simulink model "Twotanks_m71"  (R2020b)
settings: Solver=FixedStepAuto  StartTime=0.0  StopTime=300  FixedStep=0.1  RelTol=1e-3  EnableMultiTasking=on
model workspace (MAT data in the model file):
  F = [0; 0]
  Global = [3707764736; 2; 1; 1; 1; 1]
  InputSize = 5
  Operation = 'value'
  X = [1.91912110987  0.7189344389; 0.667300428728  0.319032887648; 0.539327875678  0.291550549769; 1.11428719774  0.782058235411; 0.458496889769  0.886118463221]
  cs : handle (value not decoded)
  curPath = '/Users/ceren.gebizli/Desktop/Shiva/QRA-Search/QRA-Search/Problems/SimulinkTesting'
  ext = ''
  generatedFile = '/Users/khouloud.gaaloul/Documents/Projects/SOCRaTeS/socrates/software/scalability/Simulink_Models/Twotanks/Twotanks_Model'
  hws = [3707764736; 2; 1; 1; 1; 1]
  input = [1.91912110987  0.7189344389; 0.667300428728  0.319032887648; 0.539327875678  0.291550549769; 1.11428719774  0.782058235411; 0.458496889769  0.886118463221]
  inputSize = 1
  j = 2
  m = matlab.io.MatFile
  m.Properties = matlab.io.matfile.Properties
  m.Properties.SupportsPartialAccess = 0
  m.Properties.Source = '/Users/khouloud.gaaloul/Documents/Projects/SOCRaTeS/socrates/software/scalability/RQ3/testcases/twotanks_tc_1.mat'
  matfilename = 'twotanks_tc_1.mat'
  model_cs : handle (value not decoded)
  modelpath = '/Users/khouloud.gaaloul/Documents/Projects/SOCRaTeS/socrates/software/scalability/Simulink_Models/Twotanks/'
  name = 'Twotanks_Model'
  nbrInputs = 2
  nbrTimeSteps = 5001
  p = 1
  path = '/Users/khouloud.gaaloul/Documents/Projects/SOCRaTeS/socrates/software/scalability/Simulink_Models/Twotanks'
  pr.model_name = 'Twotanks_Model'
  pr.fc = 5000
  pr.stime = 500
  problem : object (value not decoded)
  problems = {'twotanks'}
  tank1_init_height_m = 1.91912110987
  tank2_init_height_m = 0.7189344389
  testcase.signal = [0.0460270741829 0.899426437102]
  timestep = 2
  var.signal = [0.0460270741829 0.899426437102]
undefined symbols (not defined in the file): tank1_cross_section_area_m2_in, tank1_pump_flow_rate_m3s_in, tank1_sensor_hi_height_m_in, tank1_sensor_lo_height_m_in, tank1_valve_flow_rate_m3s_in, tank2_cross_section_area_m2_in, tank2_e_valve_flow_rate_m3s_in, tank2_p_valve_flow_rate_m3s_in, tank2_sensor_hi_height_m_in, tank2_sensor_lo_height_m_in, tank2_sensor_md_height_m_in
libraries: simulink x12
settings Model: Creator=Kerianne  LastModifiedBy=Xiao Ling
settings DataIOCC: ExternalInput=var  SaveFormat=StructureWithTime  SignalLoggingSaveFormat=ModelDataLogs  ReturnWorkspaceOutputs=off  OutputSaveName=varout  LoggingToFile=on
settings OptimizationCC: DefaultParameterBehavior=Inlined  ExpressionDepthLimit=2147483647  LifeSpan=inf
settings DebuggingCC: UnderspecifiedInitializationDetection=Classic  MergeDetectMultiDrivingBlocksExec=none  SolverPrmCheckMsg=warning  MultiTaskDSMMsg=warning  MultiTaskCondExecSysMsg=none  StateNameClashWarn=warning  SFUnexpectedBacktrackingDiag=warning  SFNoUnconditionalDefaultTransitionDiag=warning  SFExecutionAtInitializationDiag=none  ArithmeticOperatorsInVariantConditions=warning
settings HardwareCC: ProdBitPerPointer=32  ProdBitPerSizeT=32  ProdBitPerPtrDiffT=32  ProdLargestAtomicFloat=None  ProdIntDivRoundTo=Undefined  ProdEndianess=Unspecified  ProdWordSize=32  ProdHWDeviceType=32-bit Generic
settings ModelReferenceCC: PropagateSignalLabelsOutOfModel=off
settings SFSimCC: SimUseLocalCustomCode=off  CustomCodeUndefinedFunction=UseInterfaceOnly
settings RTWCC: RTWUseLocalCustomCode=off
settings CodeAppCC: StateflowObjectComments=on
settings GRTTargetCC: TargetLangStandard=C89/C90 (ANSI)
settings ConfigComp: CovMetricSettings=dw  CovSaveCumulativeToWorkspaceVar=on  CovSaveSingleToWorkspaceVar=on  CovExternalEMLEnable=off

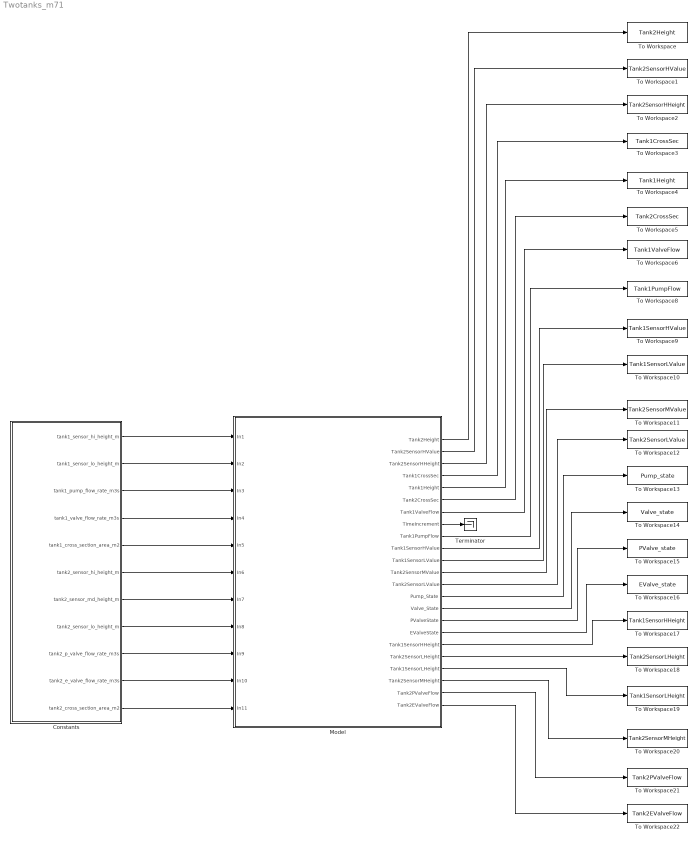
== system Twotanks_m71 ==
  Constants : Subsystem
  Model : Subsystem
  Terminator : Terminator
  To Workspace : ToWorkspace  VariableName=Tank2Height  SampleTime=-1
  To Workspace1 : ToWorkspace  VariableName=Tank2SensorHValue  SampleTime=-1
  To Workspace10 : ToWorkspace  VariableName=Tank1SensorLValue  SampleTime=-1
  To Workspace11 : ToWorkspace  VariableName=Tank2SensorMValue  SampleTime=-1
  To Workspace12 : ToWorkspace  VariableName=Tank2SensorLValue  SampleTime=-1
  To Workspace13 : ToWorkspace  VariableName=Pump_state  SampleTime=-1
  To Workspace14 : ToWorkspace  VariableName=Valve_state  SampleTime=-1
  To Workspace15 : ToWorkspace  VariableName=PValve_state  SampleTime=-1
  To Workspace16 : ToWorkspace  VariableName=EValve_state  SampleTime=-1
  To Workspace17 : ToWorkspace  VariableName=Tank1SensorHHeight  SampleTime=-1
  To Workspace18 : ToWorkspace  VariableName=Tank2SensorLHeight  SampleTime=-1
  To Workspace19 : ToWorkspace  VariableName=Tank1SensorLHeight  SampleTime=-1
  To Workspace2 : ToWorkspace  VariableName=Tank2SensorHHeight  SampleTime=-1
  To Workspace20 : ToWorkspace  VariableName=Tank2SensorMHeight  SampleTime=-1
  To Workspace21 : ToWorkspace  VariableName=Tank2PValveFlow  SampleTime=-1
  To Workspace22 : ToWorkspace  VariableName=Tank2EValveFlow  SampleTime=-1
  To Workspace3 : ToWorkspace  VariableName=Tank1CrossSec  SampleTime=-1
  To Workspace4 : ToWorkspace  VariableName=Tank1Height  SampleTime=-1
  To Workspace5 : ToWorkspace  VariableName=Tank2CrossSec  SampleTime=-1
  To Workspace6 : ToWorkspace  VariableName=Tank1ValveFlow  SampleTime=-1
  To Workspace8 : ToWorkspace  VariableName=Tank1PumpFlow  SampleTime=-1
  To Workspace9 : ToWorkspace  VariableName=Tank1SensorHValue  SampleTime=-1
  wires:
  Constants/1(tank1_sensor_hi_height_m) -> Model/1(In1)
  Constants/2(tank1_sensor_lo_height_m) -> Model/2(In2)
  Constants/3(tank1_pump_flow_rate_m3s) -> Model/3(In3)
  Constants/4(tank1_valve_flow_rate_m3s) -> Model/4(In4)
  Constants/5(tank1_cross_section_area_m2) -> Model/5(In5)
  Constants/6(tank2_sensor_hi_height_m) -> Model/6(In6)
  Constants/7(tank2_sensor_md_height_m) -> Model/7(In7)
  Constants/8(tank2_sensor_lo_height_m) -> Model/8(In8)
  Constants/9(tank2_p_valve_flow_rate_m3s) -> Model/9(In9)
  Constants/10(tank2_e_valve_flow_rate_m3s) -> Model/10(In10)
  Constants/11(tank2_cross_section_area_m2) -> Model/11(In11)
  Model/1(Tank2Height) -> To Workspace/1
  Model/2(Tank2SensorHValue) -> To Workspace1/1
  Model/3(Tank2SensorHHeight) -> To Workspace2/1
  Model/7(Tank1ValveFlow) -> To Workspace6/1
  Model/8(TimeIncrement) -> Terminator/1
  Model/6(Tank2CrossSec) -> To Workspace5/1
  Model/5(Tank1Height) -> To Workspace4/1
  Model/9(Tank1PumpFlow) -> To Workspace8/1
  Model/10(Tank1SensorHValue) -> To Workspace9/1
  Model/11(Tank1SensorLValue) -> To Workspace10/1
  Model/12(Tank2SensorMValue) -> To Workspace11/1
  Model/13(Tank2SensorLValue) -> To Workspace12/1
  Model/16(PValveState) -> To Workspace15/1
  Model/15(Valve_State) -> To Workspace14/1
  Model/14(Pump_State) -> To Workspace13/1
  Model/19(Tank2SensorLHeight) -> To Workspace18/1
  Model/18(Tank1SensorHHeight) -> To Workspace17/1
  Model/17(EValveState) -> To Workspace16/1
  Model/20(Tank1SensorLHeight) -> To Workspace19/1
  Model/21(Tank2SensorMHeight) -> To Workspace20/1
  Model/23(Tank2EValveFlow) -> To Workspace22/1
  Model/22(Tank2PValveFlow) -> To Workspace21/1
  Model/4(Tank1CrossSec) -> To Workspace3/1

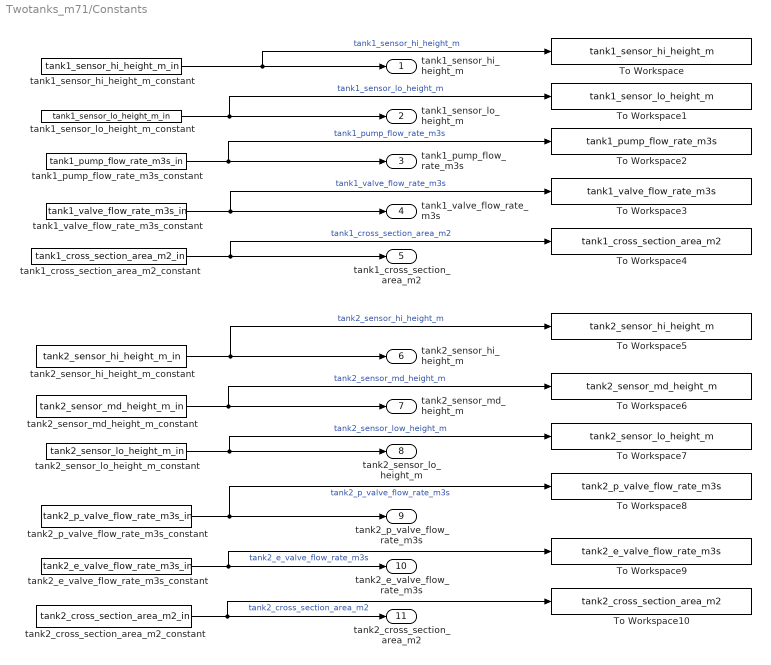
== system Twotanks_m71/Constants ==
  To Workspace : ToWorkspace  VariableName=tank1_sensor_hi_height_m  SampleTime=-1
  To Workspace1 : ToWorkspace  VariableName=tank1_sensor_lo_height_m  SampleTime=-1
  To Workspace10 : ToWorkspace  VariableName=tank2_cross_section_area_m2  SampleTime=-1
  To Workspace2 : ToWorkspace  VariableName=tank1_pump_flow_rate_m3s  SampleTime=-1
  To Workspace3 : ToWorkspace  VariableName=tank1_valve_flow_rate_m3s  SampleTime=-1
  To Workspace4 : ToWorkspace  VariableName=tank1_cross_section_area_m2  SampleTime=-1
  To Workspace5 : ToWorkspace  VariableName=tank2_sensor_hi_height_m  SampleTime=-1
  To Workspace6 : ToWorkspace  VariableName=tank2_sensor_md_height_m  SampleTime=-1
  To Workspace7 : ToWorkspace  VariableName=tank2_sensor_lo_height_m  SampleTime=-1
  To Workspace8 : ToWorkspace  VariableName=tank2_p_valve_flow_rate_m3s  SampleTime=-1
  To Workspace9 : ToWorkspace  VariableName=tank2_e_valve_flow_rate_m3s  SampleTime=-1
  tank1_cross_section_area_m2_constant : Constant  Value=tank1_cross_section_area_m2_in
  tank1_pump_flow_rate_m3s_constant : Constant  Value=tank1_pump_flow_rate_m3s_in
  tank1_sensor_hi_height_m_constant : Constant  Value=tank1_sensor_hi_height_m_in
  tank1_sensor_lo_height_m_constant : Constant  Value=tank1_sensor_lo_height_m_in
  tank1_valve_flow_rate_m3s_constant : Constant  Value=tank1_valve_flow_rate_m3s_in
  tank2_cross_section_area_m2_constant : Constant  Value=tank2_cross_section_area_m2_in
  tank2_e_valve_flow_rate_m3s_constant : Constant  Value=tank2_e_valve_flow_rate_m3s_in
  tank2_p_valve_flow_rate_m3s_constant : Constant  Value=tank2_p_valve_flow_rate_m3s_in
  tank2_sensor_hi_height_m_constant : Constant  Value=tank2_sensor_hi_height_m_in
  tank2_sensor_lo_height_m_constant : Constant  Value=tank2_sensor_lo_height_m_in
  tank2_sensor_md_height_m_constant : Constant  Value=tank2_sensor_md_height_m_in
  tank1_sensor_hi_height_m : Outport  VectorParamsAs1DForOutWhenUnconnected=off
  tank1_sensor_lo_height_m : Outport  Port=2  VectorParamsAs1DForOutWhenUnconnected=off
  tank1_pump_flow_rate_m3s : Outport  Port=3  VectorParamsAs1DForOutWhenUnconnected=off
  tank1_valve_flow_rate_m3s : Outport  Port=4  VectorParamsAs1DForOutWhenUnconnected=off
  tank1_cross_section_area_m2 : Outport  Port=5  VectorParamsAs1DForOutWhenUnconnected=off
  tank2_sensor_hi_height_m : Outport  Port=6  VectorParamsAs1DForOutWhenUnconnected=off
  tank2_sensor_md_height_m : Outport  Port=7  VectorParamsAs1DForOutWhenUnconnected=off
  tank2_sensor_lo_height_m : Outport  Port=8  VectorParamsAs1DForOutWhenUnconnected=off
  tank2_p_valve_flow_rate_m3s : Outport  Port=9  VectorParamsAs1DForOutWhenUnconnected=off
  tank2_e_valve_flow_rate_m3s : Outport  Port=10  VectorParamsAs1DForOutWhenUnconnected=off
  tank2_cross_section_area_m2 : Outport  Port=11  VectorParamsAs1DForOutWhenUnconnected=off
  wires:
  tank2_sensor_hi_height_m_constant/1 -> To Workspace5/1, tank2_sensor_hi_height_m/1  "tank2_sensor_hi_height_m"
  tank2_sensor_lo_height_m_constant/1 -> To Workspace7/1, tank2_sensor_lo_height_m/1  "tank2_sensor_low_height_m"
  tank1_sensor_hi_height_m_constant/1 -> To Workspace/1, tank1_sensor_hi_height_m/1  "tank1_sensor_hi_height_m"
  tank1_pump_flow_rate_m3s_constant/1 -> tank1_pump_flow_rate_m3s/1, To Workspace2/1  "tank1_pump_flow_rate_m3s"
  tank1_cross_section_area_m2_constant/1 -> To Workspace4/1, tank1_cross_section_area_m2/1  "tank1_cross_section_area_m2"
  tank1_valve_flow_rate_m3s_constant/1 -> To Workspace3/1, tank1_valve_flow_rate_m3s/1  "tank1_valve_flow_rate_m3s"
  tank1_sensor_lo_height_m_constant/1 -> tank1_sensor_lo_height_m/1, To Workspace1/1  "tank1_sensor_lo_height_m"
  tank2_p_valve_flow_rate_m3s_constant/1 -> tank2_p_valve_flow_rate_m3s/1, To Workspace8/1  "tank2_p_valve_flow_rate_m3s"
  tank2_cross_section_area_m2_constant/1 -> To Workspace10/1, tank2_cross_section_area_m2/1  "tank2_cross_section_area_m2"
  tank2_e_valve_flow_rate_m3s_constant/1 -> To Workspace9/1, tank2_e_valve_flow_rate_m3s/1  "tank2_e_valve_flow_rate_m3s"
  tank2_sensor_md_height_m_constant/1 -> To Workspace6/1, tank2_sensor_md_height_m/1  "tank2_sensor_md_height_m"

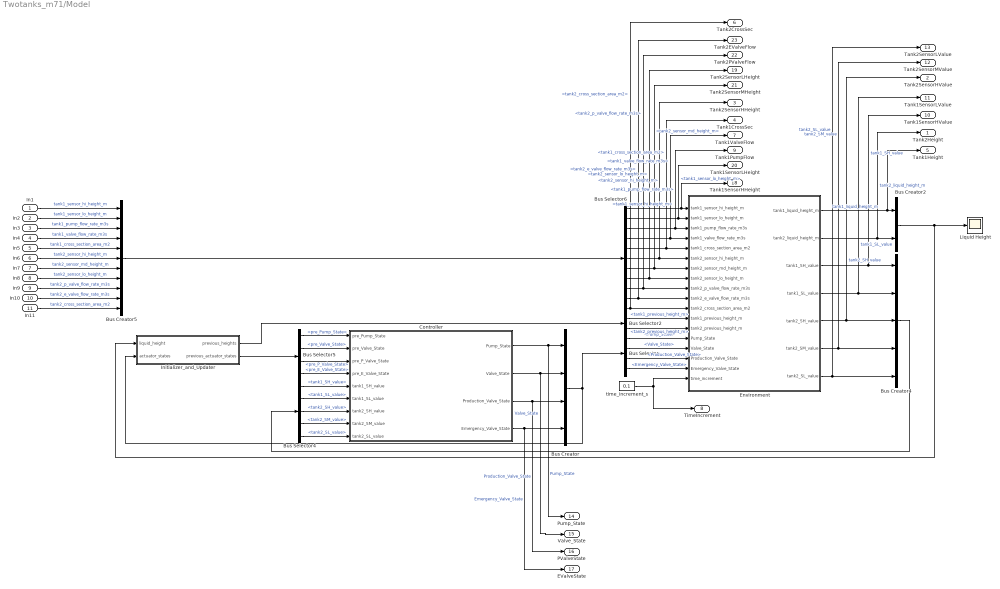
== system Twotanks_m71/Model ==
  In1 : Inport
  In2 : Inport  Port=2
  In3 : Inport  Port=3
  In4 : Inport  Port=4
  In5 : Inport  Port=5
  In6 : Inport  Port=6
  In7 : Inport  Port=7
  In8 : Inport  Port=8
  In9 : Inport  Port=9
  In10 : Inport  Port=10
  In11 : Inport  Port=11
  Bus Creator : BusCreator  Inputs=4
  Bus Creator2 : BusCreator  Inputs='tank1_liquid_height_m','tank2_liquid_height_m'
  Bus Creator4 : BusCreator  Inputs='tank1_SH_value','tank1_SL_value','tank2_SH_value','tank2_SM_value','tank2_SL_value'
  Bus Creator5 : BusCreator  Inputs='tank1_sensor_hi_height_m','tank1_sensor_lo_height_m','tank1_pump_flow_rate_m3s','tank1_valve_flow_rate_m3s','tank1_cross_section_area_m2','tank2_sensor_hi_height_m','tank2_sensor_md_height_m','tank2_sensor_lo_height_m','tank2_p_valve_flow_rate_m3s','tank2_e_valve_flow_rate_m3s','tank2_cross_section_area_m2'
  Bus Selector : BusSelector  OutputSignals=Pump_State,Valve_State,Production_Valve_State,Emergency_Valve_State
  Bus Selector2 : BusSelector  OutputSignals=tank1_previous_height_m,tank2_previous_height_m
  Bus Selector4 : BusSelector  OutputSignals=tank1_SH_value,tank1_SL_value,tank2_SH_value,tank2_SM_value,tank2_SL_value
  Bus Selector5 : BusSelector  OutputSignals=pre_Pump_State,pre_Valve_State,pre_P_Valve_State,pre_E_Valve_State
  Bus Selector6 : BusSelector  OutputSignals=tank1_sensor_hi_height_m,tank1_sensor_lo_height_m,tank1_pump_flow_rate_m3s,tank1_valve_flow_rate_m3s,tank1_cross_section_area_m2,tank2_sensor_hi_height_m,tank2_sensor_md_height_m,tank2_sensor_lo_height_m,tank2_p_valve_flow_rate_m3s,tank2_e_valve_flow_rate_m3s,tank2_cross_section_area_m2
  Controller : Subsystem
  Environment : Subsystem
  Initializer_and_Updater : Subsystem
  Liquid Height : Scope
  time_increment_s : Constant  Value=0.1
  Tank2Height : Outport  VectorParamsAs1DForOutWhenUnconnected=off
  Tank2SensorHValue : Outport  Port=2  VectorParamsAs1DForOutWhenUnconnected=off
  Tank2SensorHHeight : Outport  Port=3  VectorParamsAs1DForOutWhenUnconnected=off
  Tank1CrossSec : Outport  Port=4  VectorParamsAs1DForOutWhenUnconnected=off
  Tank1Height : Outport  Port=5  VectorParamsAs1DForOutWhenUnconnected=off
  Tank2CrossSec : Outport  Port=6  VectorParamsAs1DForOutWhenUnconnected=off
  Tank1ValveFlow : Outport  Port=7  VectorParamsAs1DForOutWhenUnconnected=off
  TimeIncrement : Outport  Port=8  VectorParamsAs1DForOutWhenUnconnected=off
  Tank1PumpFlow : Outport  Port=9  VectorParamsAs1DForOutWhenUnconnected=off
  Tank1SensorHValue : Outport  Port=10  VectorParamsAs1DForOutWhenUnconnected=off
  Tank1SensorLValue : Outport  Port=11  VectorParamsAs1DForOutWhenUnconnected=off
  Tank2SensorMValue : Outport  Port=12  VectorParamsAs1DForOutWhenUnconnected=off
  Tank2SensorLValue : Outport  Port=13  VectorParamsAs1DForOutWhenUnconnected=off
  Pump_State : Outport  Port=14  VectorParamsAs1DForOutWhenUnconnected=off
  Valve_State : Outport  Port=15  VectorParamsAs1DForOutWhenUnconnected=off
  PValveState : Outport  Port=16  VectorParamsAs1DForOutWhenUnconnected=off
  EValveState : Outport  Port=17  VectorParamsAs1DForOutWhenUnconnected=off
  Tank1SensorHHeight : Outport  Port=18  VectorParamsAs1DForOutWhenUnconnected=off
  Tank2SensorLHeight : Outport  Port=19  VectorParamsAs1DForOutWhenUnconnected=off
  Tank1SensorLHeight : Outport  Port=20  VectorParamsAs1DForOutWhenUnconnected=off
  Tank2SensorMHeight : Outport  Port=21  VectorParamsAs1DForOutWhenUnconnected=off
  Tank2PValveFlow : Outport  Port=22  VectorParamsAs1DForOutWhenUnconnected=off
  Tank2EValveFlow : Outport  Port=23  VectorParamsAs1DForOutWhenUnconnected=off
  wires:
  In8/1 -> Bus Creator5/8  "tank2_sensor_lo_height_m"
  Bus Selector6/7 -> Environment/7(tank2_sensor_md_height_m), Tank2SensorMHeight/1  "<tank2_sensor_md_height_m>"
  Initializer_and_Updater/1(previous_heights) -> Bus Selector2/1
  Bus Selector6/10 -> Environment/10(tank2_e_valve_flow_rate_m3s), Tank2EValveFlow/1  "<tank2_e_valve_flow_rate_m3s>"
  Bus Selector6/3 -> Tank1PumpFlow/1, Environment/3(tank1_pump_flow_rate_m3s)  "<tank1_pump_flow_rate_m3s>"
  Bus Selector5/1 -> Controller/1(pre_Pump_State)  "<pre_Pump_State>"
  Environment/1(tank1_liquid_height_m) -> Tank1Height/1, Bus Creator2/1  "tank1_liquid_height_m"
  Bus Selector6/1 -> Tank1SensorHHeight/1, Environment/1(tank1_sensor_hi_height_m)  "<tank1_sensor_hi_height_m>"
  Bus Selector4/3 -> Controller/7(tank2_SH_value)  "<tank2_SH_value>"
  Bus Selector5/3 -> Controller/3(pre_P_Valve_State)  "<pre_P_Valve_State>"
  Bus Selector4/2 -> Controller/6(tank1_SL_value)  "<tank1_SL_value>"
  In6/1 -> Bus Creator5/6  "tank2_sensor_hi_height_m"
  Bus Selector/2 -> Environment/15(Valve_State)  "<Valve_State>"
  time_increment_s/1 -> Environment/18(time_increment), TimeIncrement/1
  Bus Selector6/6 -> Tank2SensorHHeight/1, Environment/6(tank2_sensor_hi_height_m)  "<tank2_sensor_hi_height_m>"
  Bus Selector4/4 -> Controller/8(tank2_SM_value)  "<tank2_SM_value>"
  In1/1 -> Bus Creator5/1  "tank1_sensor_hi_height_m"
  Environment/6(tank2_SM_value) -> Bus Creator4/4, Tank2SensorMValue/1  "tank2_SM_value"
  In7/1 -> Bus Creator5/7  "tank2_sensor_md_height_m"
  Bus Selector4/1 -> Controller/5(tank1_SH_value)  "<tank1_SH_value>"
  Controller/4(Emergency_Valve_State) -> EValveState/1, Bus Creator/4  "Emergency_Valve_State"
  Bus Selector6/9 -> Environment/9(tank2_p_valve_flow_rate_m3s), Tank2PValveFlow/1  "<tank2_p_valve_flow_rate_m3s>"
  Bus Selector6/4 -> Environment/4(tank1_valve_flow_rate_m3s), Tank1ValveFlow/1  "<tank1_valve_flow_rate_m3s>"
  Bus Creator5/1 -> Bus Selector6/1
  In5/1 -> Bus Creator5/5  "tank1_cross_section_area_m2"
  In10/1 -> Bus Creator5/10  "tank2_e_valve_flow_rate_m3s"
  Bus Creator4/1 -> Bus Selector4/1
  Environment/2(tank2_liquid_height_m) -> Tank2Height/1, Bus Creator2/2  "tank2_liquid_height_m"
  Bus Selector6/8 -> Environment/8(tank2_sensor_lo_height_m), Tank2SensorLHeight/1  "<tank2_sensor_lo_height_m>"
  Bus Selector/4 -> Environment/17(Emergency_Valve_State)  "<Emergency_Valve_State>"
  Environment/4(tank1_SL_value) -> Bus Creator4/2, Tank1SensorLValue/1  "tank1_SL_value"
  Bus Selector/3 -> Environment/16(Production_Valve_State)  "<Production_Valve_State>"
  In2/1 -> Bus Creator5/2  "tank1_sensor_lo_height_m"
  Bus Selector4/5 -> Controller/9(tank2_SL_value)  "<tank2_SL_value>"
  Bus Selector/1 -> Environment/14(Pump_State)  "<Pump_State>"
  Bus Selector6/2 -> Environment/2(tank1_sensor_lo_height_m), Tank1SensorLHeight/1  "<tank1_sensor_lo_height_m>"
  Bus Selector6/5 -> Tank1CrossSec/1, Environment/5(tank1_cross_section_area_m2)  "<tank1_cross_section_area_m2>"
  Environment/3(tank1_SH_value) -> Tank1SensorHValue/1, Bus Creator4/1  "tank1_SH_value"
  Controller/2(Valve_State) -> Bus Creator/2, Valve_State/1  "Valve_State"
  In4/1 -> Bus Creator5/4  "tank1_valve_flow_rate_m3s"
  In11/1 -> Bus Creator5/11  "tank2_cross_section_area_m2"
  Initializer_and_Updater/2(previous_actuator_states) -> Bus Selector5/1
  Environment/5(tank2_SH_value) -> Bus Creator4/3, Tank2SensorHValue/1  "tank2_SH_value"
  Bus Selector5/2 -> Controller/2(pre_Valve_State)  "<pre_Valve_State>"
  Bus Selector2/1 -> Environment/12(tank1_previous_height_m)  "<tank1_previous_height_m>"
  Environment/7(tank2_SL_value) -> Bus Creator4/5, Tank2SensorLValue/1  "tank2_SL_value"
  Controller/3(Production_Valve_State) -> PValveState/1, Bus Creator/3  "Production_Valve_State"
  Controller/1(Pump_State) -> Bus Creator/1, Pump_State/1  "Pump_State"
  In3/1 -> Bus Creator5/3  "tank1_pump_flow_rate_m3s"
  Bus Creator/1 -> Bus Selector/1, Initializer_and_Updater/2(actuator_states)
  Bus Creator2/1 -> Initializer_and_Updater/1(liquid_height), Liquid Height/1
  Bus Selector6/11 -> Environment/11(tank2_cross_section_area_m2), Tank2CrossSec/1  "<tank2_cross_section_area_m2>"
  Bus Selector2/2 -> Environment/13(tank2_previous_height_m)  "<tank2_previous_height_m>"
  Bus Selector5/4 -> Controller/4(pre_E_Valve_State)  "<pre_E_Valve_State>"
  In9/1 -> Bus Creator5/9  "tank2_p_valve_flow_rate_m3s"

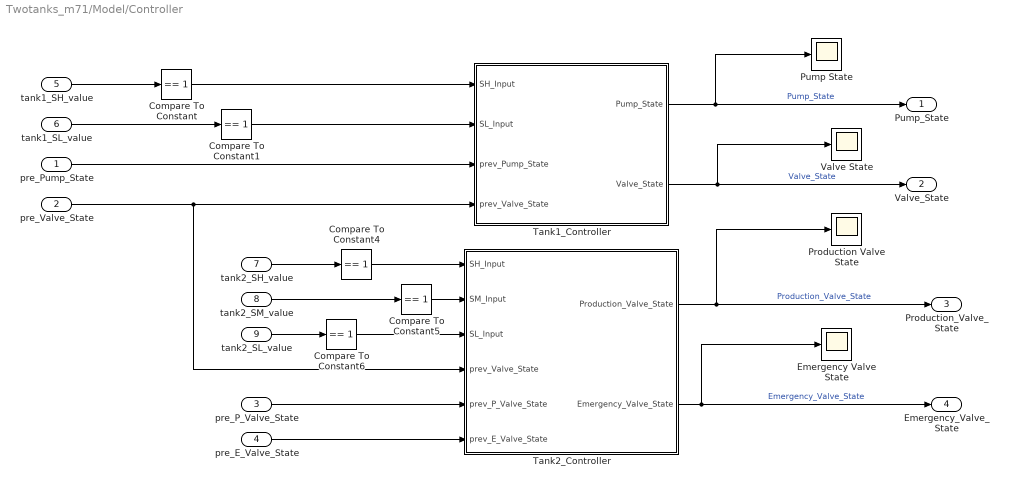
== system Twotanks_m71/Model/Controller ==
  pre_Pump_State : Inport
  pre_Valve_State : Inport  Port=2
  pre_P_Valve_State : Inport  Port=3
  pre_E_Valve_State : Inport  Port=4
  tank1_SH_value : Inport  Port=5
  tank1_SL_value : Inport  Port=6
  tank2_SH_value : Inport  Port=7
  tank2_SM_value : Inport  Port=8
  tank2_SL_value : Inport  Port=9
  Compare To Constant{,1,4..6} (5 alike) : simulink/Logic and Bit Operations/Compare To Constant  relop===  const=1  OutDataTypeStr=boolean
  Emergency Valve State : Scope
  Production Valve State : Scope
  "Pump State " : Scope
  Tank1_Controller : Subsystem
  Tank2_Controller : Subsystem
  Valve State : Scope
  Pump_State : Outport  VectorParamsAs1DForOutWhenUnconnected=off
  Valve_State : Outport  Port=2  VectorParamsAs1DForOutWhenUnconnected=off
  Production_Valve_State : Outport  Port=3  VectorParamsAs1DForOutWhenUnconnected=off
  Emergency_Valve_State : Outport  Port=4  VectorParamsAs1DForOutWhenUnconnected=off
  wires:
  tank1_SL_value/1 -> Compare To Constant1/1
  tank2_SL_value/1 -> Compare To Constant6/1
  pre_E_Valve_State/1 -> Tank2_Controller/6(prev_E_Valve_State)
  Compare To Constant1/1 -> Tank1_Controller/2(SL_Input)
  Tank1_Controller/1(Pump_State) -> Pump_State/1, "Pump State "/1  "Pump_State"
  Tank1_Controller/2(Valve_State) -> Valve_State/1, Valve State/1  "Valve_State"
  Compare To Constant/1 -> Tank1_Controller/1(SH_Input)
  pre_Pump_State/1 -> Tank1_Controller/3(prev_Pump_State)
  tank2_SH_value/1 -> Compare To Constant4/1
  Compare To Constant6/1 -> Tank2_Controller/3(SL_Input)
  Compare To Constant4/1 -> Tank2_Controller/1(SH_Input)
  tank1_SH_value/1 -> Compare To Constant/1
  pre_Valve_State/1 -> Tank2_Controller/4(prev_Valve_State), Tank1_Controller/4(prev_Valve_State)
  Tank2_Controller/2(Emergency_Valve_State) -> Emergency_Valve_State/1, Emergency Valve State/1  "Emergency_Valve_State"
  tank2_SM_value/1 -> Compare To Constant5/1
  Compare To Constant5/1 -> Tank2_Controller/2(SM_Input)
  Tank2_Controller/1(Production_Valve_State) -> Production_Valve_State/1, Production Valve State/1  "Production_Valve_State"
  pre_P_Valve_State/1 -> Tank2_Controller/5(prev_P_Valve_State)

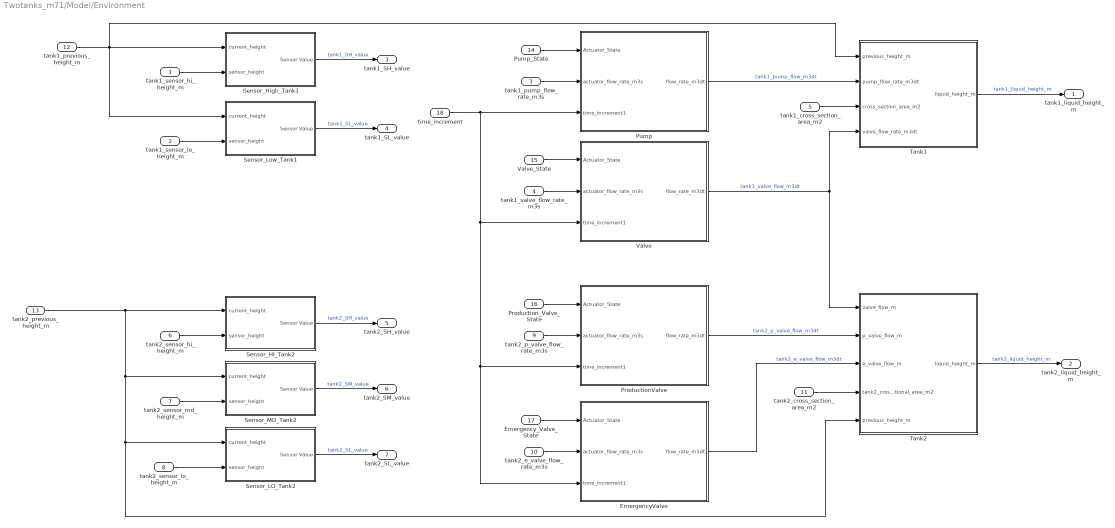
== system Twotanks_m71/Model/Environment ==
  tank1_sensor_hi_height_m : Inport
  tank1_sensor_lo_height_m : Inport  Port=2
  tank1_pump_flow_rate_m3s : Inport  Port=3
  tank1_valve_flow_rate_m3s : Inport  Port=4
  tank1_cross_section_area_m2 : Inport  Port=5
  tank2_sensor_hi_height_m : Inport  Port=6
  tank2_sensor_md_height_m : Inport  Port=7
  tank2_sensor_lo_height_m : Inport  Port=8
  tank2_p_valve_flow_rate_m3s : Inport  Port=9
  tank2_e_valve_flow_rate_m3s : Inport  Port=10
  tank2_cross_section_area_m2 : Inport  Port=11
  tank1_previous_height_m : Inport  Port=12
  tank2_previous_height_m : Inport  Port=13
  Pump_State : Inport  Port=14
  Valve_State : Inport  Port=15
  Production_Valve_State : Inport  Port=16
  Emergency_Valve_State : Inport  Port=17
  time_increment : Inport  Port=18
  EmergencyValve : Subsystem
  ProductionValve : Subsystem
  Pump : Subsystem
  Sensor_HI_Tank2 : Subsystem
  Sensor_High_Tank1 : Subsystem
  Sensor_LO_Tank2 : Subsystem
  Sensor_Low_Tank1 : Subsystem
  Sensor_MD_Tank2 : Subsystem
  Tank1 : Subsystem
  Tank2 : Subsystem
  Valve : Subsystem
  tank1_liquid_height_m : Outport  VectorParamsAs1DForOutWhenUnconnected=off
  tank2_liquid_height_m : Outport  Port=2  VectorParamsAs1DForOutWhenUnconnected=off
  tank1_SH_value : Outport  Port=3  VectorParamsAs1DForOutWhenUnconnected=off
  tank1_SL_value : Outport  Port=4  VectorParamsAs1DForOutWhenUnconnected=off
  tank2_SH_value : Outport  Port=5  VectorParamsAs1DForOutWhenUnconnected=off
  tank2_SM_value : Outport  Port=6  VectorParamsAs1DForOutWhenUnconnected=off
  tank2_SL_value : Outport  Port=7  VectorParamsAs1DForOutWhenUnconnected=off
  wires:
  Tank1/1(liquid_height_m) -> tank1_liquid_height_m/1  "tank1_liquid_height_m"
  time_increment/1 -> Pump/3(time_increment1), Valve/3(time_increment1), EmergencyValve/3(time_increment1), ProductionValve/3(time_increment1)
  tank2_sensor_hi_height_m/1 -> Sensor_HI_Tank2/2(sensor_height)
  Sensor_Low_Tank1/1(Sensor Value) -> tank1_SL_value/1  "tank1_SL_value"
  Sensor_HI_Tank2/1(Sensor Value) -> tank2_SH_value/1  "tank2_SH_value"
  Sensor_High_Tank1/1(Sensor Value) -> tank1_SH_value/1  "tank1_SH_value"
  tank1_pump_flow_rate_m3s/1 -> Pump/2(actuator_flow_rate_m3s)
  Sensor_LO_Tank2/1(Sensor Value) -> tank2_SL_value/1  "tank2_SL_value"
  tank2_sensor_lo_height_m/1 -> Sensor_LO_Tank2/2(sensor_height)
  tank1_valve_flow_rate_m3s/1 -> Valve/2(actuator_flow_rate_m3s)
  Sensor_MD_Tank2/1(Sensor Value) -> tank2_SM_value/1  "tank2_SM_value"
  tank2_p_valve_flow_rate_m3s/1 -> ProductionValve/2(actuator_flow_rate_m3s)
  tank2_previous_height_m/1 -> Sensor_HI_Tank2/1(current_height), Sensor_MD_Tank2/1(current_height), Sensor_LO_Tank2/1(current_height), Tank2/5(previous_height_m)
  EmergencyValve/1(flow_rate_m3dt) -> Tank2/3(e_valve_flow_m)  "tank2_e_valve_flow_m3dt"
  Pump/1(flow_rate_m3dt) -> Tank1/2(pump_flow_rate_m3dt)  "tank1_pump_flow_m3dt"
  Valve/1(flow_rate_m3dt) -> Tank2/1(valve_flow_m), Tank1/4(valve_flow_rate_m3dt)  "tank1_valve_flow_m3dt"
  ProductionValve/1(flow_rate_m3dt) -> Tank2/2(p_valve_flow_m)  "tank2_p_valve_flow_m3dt"
  tank2_e_valve_flow_rate_m3s/1 -> EmergencyValve/2(actuator_flow_rate_m3s)
  Valve_State/1 -> Valve/1(Actuator_State)
  Emergency_Valve_State/1 -> EmergencyValve/1(Actuator_State)
  Pump_State/1 -> Pump/1(Actuator_State)
  tank1_sensor_lo_height_m/1 -> Sensor_Low_Tank1/2(sensor_height)
  tank1_sensor_hi_height_m/1 -> Sensor_High_Tank1/2(sensor_height)
  Production_Valve_State/1 -> ProductionValve/1(Actuator_State)
  tank1_previous_height_m/1 -> Sensor_High_Tank1/1(current_height), Tank1/1(previous_height_m), Sensor_Low_Tank1/1(current_height)
  Tank2/1(liquid_height_m) -> tank2_liquid_height_m/1  "tank2_liquid_height_m"
  tank1_cross_section_area_m2/1 -> Tank1/3(cross_section_area_m2)
  tank2_cross_section_area_m2/1 -> Tank2/4(tank2_cross_sectional_area_m2)
  tank2_sensor_md_height_m/1 -> Sensor_MD_Tank2/2(sensor_height)

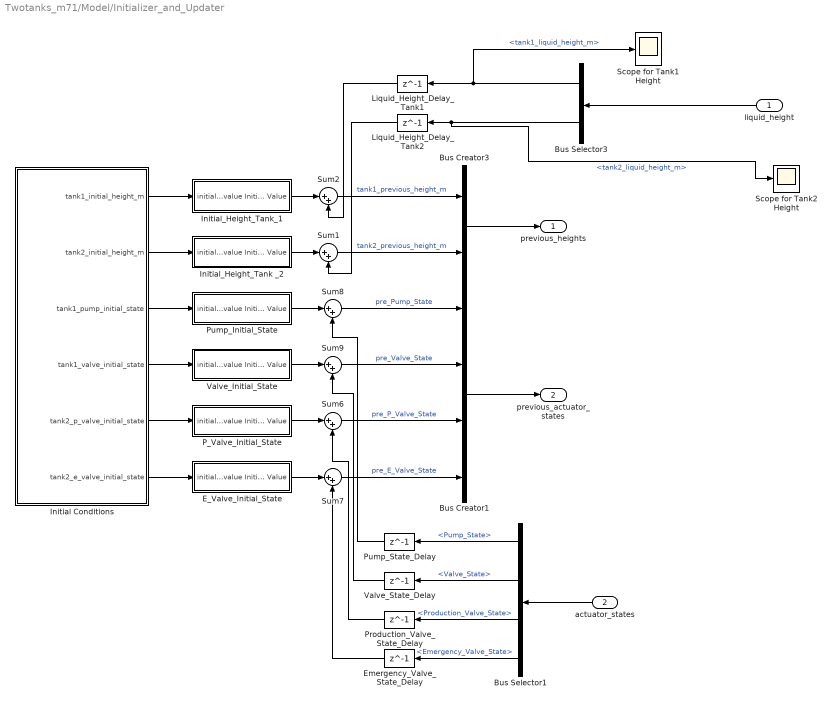
== system Twotanks_m71/Model/Initializer_and_Updater ==
  liquid_height : Inport
  actuator_states : Inport  Port=2
  Bus Creator1 : BusCreator  Inputs='pre_Pump_State','pre_Valve_State','pre_P_Valve_State','pre_E_Valve_State'
  Bus Creator3 : BusCreator  Inputs='tank1_previous_height_m','tank2_previous_height_m'
  Bus Selector1 : BusSelector  OutputSignals=Pump_State,Valve_State,Production_Valve_State,Emergency_Valve_State
  Bus Selector3 : BusSelector  OutputSignals=tank1_liquid_height_m,tank2_liquid_height_m
  E_Valve_Initial_State : Subsystem
  Emergency_Valve_State_Delay : Delay  DelayLength=1  InitialCondition=0
  Initial Conditions : Subsystem
  Initial_Height_Tank _2 : Subsystem
  Initial_Height_Tank_1 : Subsystem
  Liquid_Height_Delay_Tank1 : Delay  DelayLength=1  InitialCondition=0
  Liquid_Height_Delay_Tank2 : Delay  DelayLength=1  InitialCondition=0
  P_Valve_Initial_State : Subsystem
  Production_Valve_State_Delay : Delay  DelayLength=1  InitialCondition=0
  Pump_Initial_State : Subsystem
  Pump_State_Delay : Delay  DelayLength=1  InitialCondition=0
  "Scope for Tank1 Height " : Scope
  Scope for Tank2 Height : Scope
  Sum{1..2,6..9} (6 alike) : Sum  Inputs=|++
  Valve_Initial_State : Subsystem
  Valve_State_Delay : Delay  DelayLength=1  InitialCondition=0
  previous_heights : Outport  VectorParamsAs1DForOutWhenUnconnected=off
  previous_actuator_states : Outport  Port=2  VectorParamsAs1DForOutWhenUnconnected=off
  wires:
  Production_Valve_State_Delay/1 -> Sum6/2
  Liquid_Height_Delay_Tank1/1 -> Sum2/2
  Pump_Initial_State/1(Initial Value) -> Sum8/1
  Liquid_Height_Delay_Tank2/1 -> Sum1/2
  Valve_Initial_State/1(Initial Value) -> Sum9/1
  E_Valve_Initial_State/1(Initial Value) -> Sum7/1
  Emergency_Valve_State_Delay/1 -> Sum7/2
  Bus Selector1/3 -> Production_Valve_State_Delay/1  "<Production_Valve_State>"
  Bus Selector1/1 -> Pump_State_Delay/1  "<Pump_State>"
  Bus Selector1/2 -> Valve_State_Delay/1  "<Valve_State>"
  Bus Selector1/4 -> Emergency_Valve_State_Delay/1  "<Emergency_Valve_State>"
  Initial_Height_Tank_1/1(Initial Value) -> Sum2/1
  Initial Conditions/3(tank1_pump_initial_state) -> Pump_Initial_State/1(initial_value)
  Initial Conditions/4(tank1_valve_initial_state) -> Valve_Initial_State/1(initial_value)
  Initial Conditions/1(tank1_initial_height_m) -> Initial_Height_Tank_1/1(initial_value)
  Initial Conditions/2(tank2_initial_height_m) -> Initial_Height_Tank _2/1(initial_value)
  Initial Conditions/5(tank2_p_valve_initial_state) -> P_Valve_Initial_State/1(initial_value)
  Initial Conditions/6(tank2_e_valve_initial_state) -> E_Valve_Initial_State/1(initial_value)
  P_Valve_Initial_State/1(Initial Value) -> Sum6/1
  Sum7/1 -> Bus Creator1/4  "pre_E_Valve_State"
  Bus Selector3/2 -> Scope for Tank2 Height/1, Liquid_Height_Delay_Tank2/1  "<tank2_liquid_height_m>"
  Bus Selector3/1 -> "Scope for Tank1 Height "/1, Liquid_Height_Delay_Tank1/1  "<tank1_liquid_height_m>"
  Bus Creator3/1 -> previous_heights/1
  Sum6/1 -> Bus Creator1/3  "pre_P_Valve_State"
  Sum2/1 -> Bus Creator3/1  "tank1_previous_height_m"
  Sum9/1 -> Bus Creator1/2  "pre_Valve_State"
  Sum8/1 -> Bus Creator1/1  "pre_Pump_State"
  Sum1/1 -> Bus Creator3/2  "tank2_previous_height_m"
  Valve_State_Delay/1 -> Sum9/2
  Pump_State_Delay/1 -> Sum8/2
  Bus Creator1/1 -> previous_actuator_states/1
  liquid_height/1 -> Bus Selector3/1
  actuator_states/1 -> Bus Selector1/1
  Initial_Height_Tank _2/1(Initial Value) -> Sum1/1

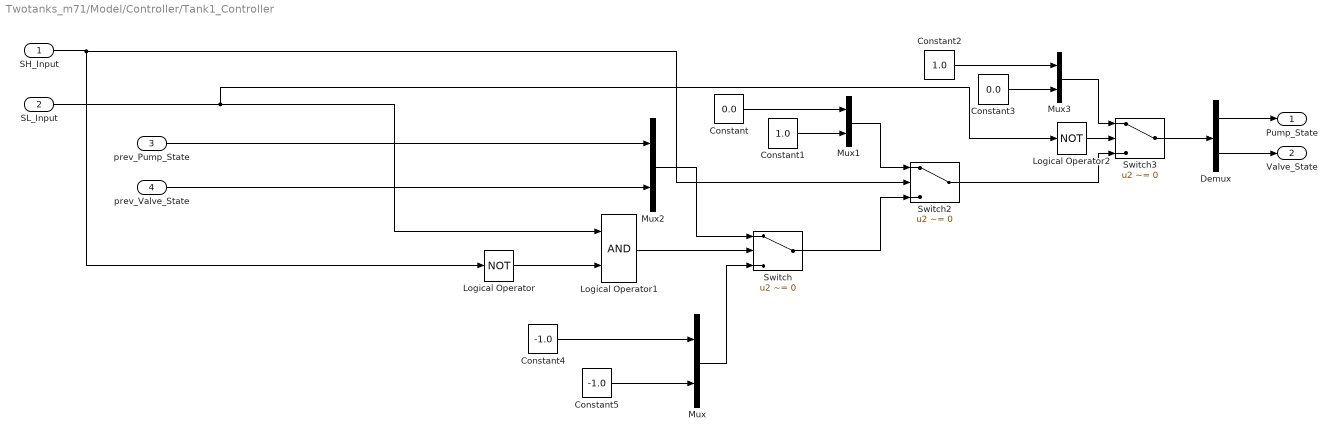
== system Twotanks_m71/Model/Controller/Tank1_Controller ==
  SH_Input : Inport
  SL_Input : Inport  Port=2
  prev_Pump_State : Inport  Port=3
  prev_Valve_State : Inport  Port=4
  Constant : Constant  Value=0.0
  Constant1 : Constant  Value=1.0
  Constant2 : Constant  Value=1.0
  Constant3 : Constant  Value=0.0
  Constant4 : Constant  Value=-1.0
  Constant5 : Constant  Value=-1.0
  Demux : Demux  Outputs=2
  Logical Operator : Logic  Operator=NOT  AllPortsSameDT=off  OutDataTypeStr=boolean
  Logical Operator1 : Logic  AllPortsSameDT=off  OutDataTypeStr=boolean
  Logical Operator2 : Logic  Operator=NOT  AllPortsSameDT=off  OutDataTypeStr=boolean
  Mux{,1..3} (4 alike) : Mux  Inputs=2
  Switch : Switch  Criteria=u2 ~= 0
  Switch2 : Switch  Criteria=u2 ~= 0
  Switch3 : Switch  Criteria=u2 ~= 0
  Pump_State : Outport  VectorParamsAs1DForOutWhenUnconnected=off
  Valve_State : Outport  Port=2  VectorParamsAs1DForOutWhenUnconnected=off
  wires:
  Mux/1 -> Switch/3
  Constant/1 -> Mux1/1
  Constant1/1 -> Mux1/2
  prev_Pump_State/1 -> Mux2/1
  prev_Valve_State/1 -> Mux2/2
  Mux2/1 -> Switch/1
  Logical Operator1/1 -> Switch/2
  Logical Operator/1 -> Logical Operator1/2
  SH_Input/1 -> Switch2/2, Logical Operator/1
  Switch/1 -> Switch2/3
  Mux1/1 -> Switch2/1
  SL_Input/1 -> Logical Operator2/1, Logical Operator1/1
  Constant2/1 -> Mux3/1
  Constant3/1 -> Mux3/2
  Mux3/1 -> Switch3/1
  Switch3/1 -> Demux/1
  Demux/2 -> Valve_State/1
  Logical Operator2/1 -> Switch3/2
  Constant4/1 -> Mux/1
  Constant5/1 -> Mux/2
  Demux/1 -> Pump_State/1
  Switch2/1 -> Switch3/3

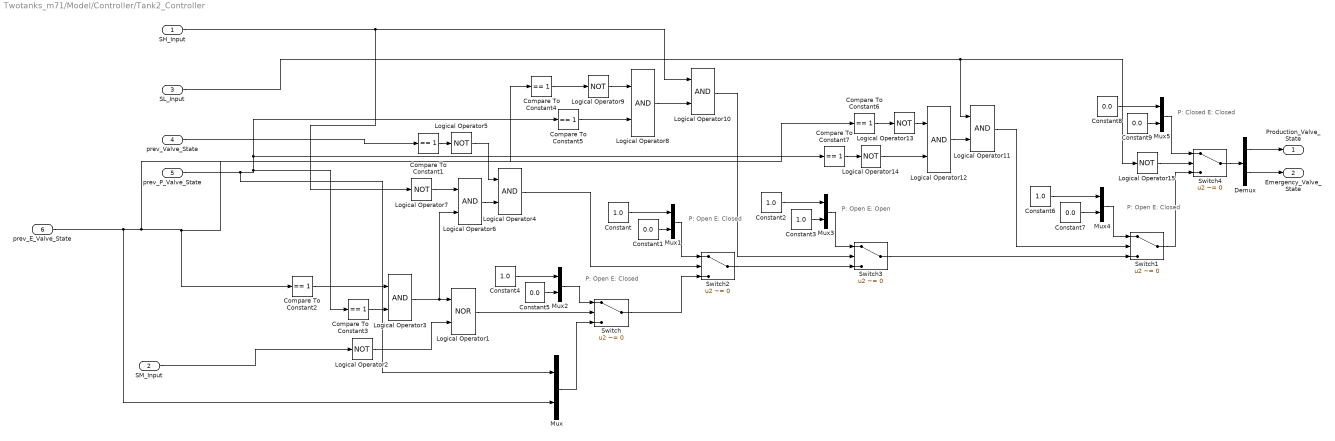
== system Twotanks_m71/Model/Controller/Tank2_Controller ==
  note: P: Open
      | E: Closed
  note: P: Open
      | E: Closed
  note: P: Open
      | E: Open
  note: P: Open
      | E: Closed
  note: P: Closed
      | E: Closed
  SH_Input : Inport
  SM_Input : Inport  Port=2
  SL_Input : Inport  Port=3
  prev_Valve_State : Inport  Port=4
  prev_P_Valve_State : Inport  Port=5
  prev_E_Valve_State : Inport  Port=6
  Compare To Constant{1..7} (7 alike) : simulink/Logic and Bit Operations/Compare To Constant  relop===  const=1  OutDataTypeStr=boolean
  Constant{,2..4,6} (5 alike) : Constant  Value=1.0
  Constant{1,5,7..9} (5 alike) : Constant  Value=0.0
  Demux : Demux  Outputs=2
  Logical Operator1 : Logic  Operator=NOR  AllPortsSameDT=off  OutDataTypeStr=boolean
  Logical Operator{3..4,6,8,10..12} (7 alike) : Logic  AllPortsSameDT=off  OutDataTypeStr=boolean
  Logical Operator{2,5,7,9,13..15} (7 alike) : Logic  Operator=NOT  AllPortsSameDT=off  OutDataTypeStr=boolean
  Mux{,1..5} (6 alike) : Mux  Inputs=2
  Switch{,1..4} (5 alike) : Switch  Criteria=u2 ~= 0
  Production_Valve_State : Outport  VectorParamsAs1DForOutWhenUnconnected=off
  Emergency_Valve_State : Outport  Port=2  VectorParamsAs1DForOutWhenUnconnected=off
  wires:
  prev_P_Valve_State/1 -> Mux/1, Compare To Constant3/1, Compare To Constant7/1, Compare To Constant5/1
  Mux/1 -> Switch/3
  Constant/1 -> Mux1/1
  Constant1/1 -> Mux1/2
  Logical Operator1/1 -> Switch/2
  SM_Input/1 -> Logical Operator2/1
  Switch/1 -> Switch2/3
  Logical Operator4/1 -> Switch2/2
  Mux1/1 -> Switch2/1
  Switch2/1 -> Switch3/3
  Logical Operator10/1 -> Switch3/2
  Demux/1 -> Production_Valve_State/1
  Demux/2 -> Emergency_Valve_State/1
  prev_Valve_State/1 -> Compare To Constant1/1
  Logical Operator5/1 -> Logical Operator4/1
  Logical Operator6/1 -> Logical Operator4/2
  Logical Operator3/1 -> Logical Operator6/2, Logical Operator1/1
  Logical Operator2/1 -> Logical Operator1/2
  SH_Input/1 -> Logical Operator7/1, Logical Operator10/1
  Logical Operator7/1 -> Logical Operator6/1
  Constant4/1 -> Mux2/1
  Constant5/1 -> Mux2/2
  Mux2/1 -> Switch/1
  Logical Operator9/1 -> Logical Operator8/1
  Logical Operator8/1 -> Logical Operator10/2
  Constant2/1 -> Mux3/1
  Constant3/1 -> Mux3/2
  Mux3/1 -> Switch3/1
  prev_E_Valve_State/1 -> Mux/2, Compare To Constant4/1, Compare To Constant6/1, Compare To Constant2/1
  Logical Operator13/1 -> Logical Operator12/1
  Logical Operator12/1 -> Logical Operator11/2
  Logical Operator14/1 -> Logical Operator12/2
  Switch3/1 -> Switch1/3
  Logical Operator11/1 -> Switch1/2
  Constant6/1 -> Mux4/1
  Constant7/1 -> Mux4/2
  Mux4/1 -> Switch1/1
  Switch1/1 -> Switch4/3
  Logical Operator15/1 -> Switch4/2
  SL_Input/1 -> Logical Operator15/1, Logical Operator11/1
  Switch4/1 -> Demux/1
  Constant8/1 -> Mux5/1
  Constant9/1 -> Mux5/2
  Mux5/1 -> Switch4/1
  Compare To Constant1/1 -> Logical Operator5/1
  Compare To Constant2/1 -> Logical Operator3/1
  Compare To Constant3/1 -> Logical Operator3/2
  Compare To Constant4/1 -> Logical Operator9/1
  Compare To Constant5/1 -> Logical Operator8/2
  Compare To Constant6/1 -> Logical Operator13/1
  Compare To Constant7/1 -> Logical Operator14/1

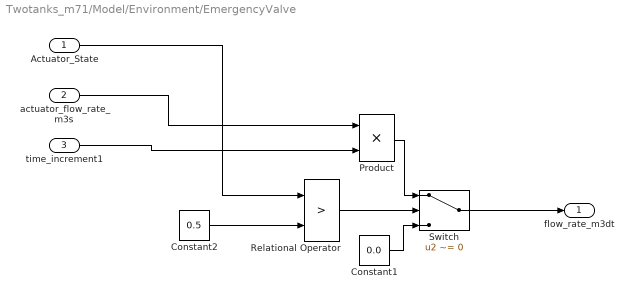
== system Twotanks_m71/Model/Environment/EmergencyValve ==
  Actuator_State : Inport
  actuator_flow_rate_m3s : Inport  Port=2
  time_increment1 : Inport  Port=3
  Constant1 : Constant  Value=0.0
  Constant2 : Constant  Value=0.5
  Product : Product
  Relational Operator : RelationalOperator  Operator=>  OutDataTypeStr=boolean  RndMeth=Nearest
  Switch : Switch  Criteria=u2 ~= 0
  flow_rate_m3dt : Outport  VectorParamsAs1DForOutWhenUnconnected=off
  wires:
  Relational Operator/1 -> Switch/2
  Actuator_State/1 -> Relational Operator/1
  time_increment1/1 -> Product/2
  Constant1/1 -> Switch/3
  Constant2/1 -> Relational Operator/2
  Switch/1 -> flow_rate_m3dt/1
  Product/1 -> Switch/1
  actuator_flow_rate_m3s/1 -> Product/1

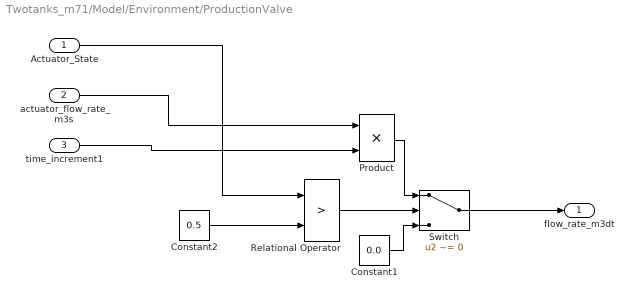
== system Twotanks_m71/Model/Environment/ProductionValve ==
  Actuator_State : Inport
  actuator_flow_rate_m3s : Inport  Port=2
  time_increment1 : Inport  Port=3
  Constant1 : Constant  Value=0.0
  Constant2 : Constant  Value=0.5
  Product : Product
  Relational Operator : RelationalOperator  Operator=>  OutDataTypeStr=boolean  RndMeth=Nearest
  Switch : Switch  Criteria=u2 ~= 0
  flow_rate_m3dt : Outport  VectorParamsAs1DForOutWhenUnconnected=off
  wires:
  actuator_flow_rate_m3s/1 -> Product/1
  Product/1 -> Switch/1
  Switch/1 -> flow_rate_m3dt/1
  Constant2/1 -> Relational Operator/2
  Constant1/1 -> Switch/3
  time_increment1/1 -> Product/2
  Actuator_State/1 -> Relational Operator/1
  Relational Operator/1 -> Switch/2

== system Twotanks_m71/Model/Environment/Pump ==
  Actuator_State : Inport
  actuator_flow_rate_m3s : Inport  Port=2
  time_increment1 : Inport  Port=3
  Constant1 : Constant  Value=0.0
  Constant2 : Constant  Value=0.5
  Product : Product
  Relational Operator : RelationalOperator  Operator=>  OutDataTypeStr=boolean  RndMeth=Nearest
  Switch : Switch  Criteria=u2 ~= 0
  flow_rate_m3dt : Outport  VectorParamsAs1DForOutWhenUnconnected=off
  wires:
  actuator_flow_rate_m3s/1 -> Product/1
  Product/1 -> Switch/1
  Switch/1 -> flow_rate_m3dt/1
  Constant2/1 -> Relational Operator/2
  Constant1/1 -> Switch/3
  time_increment1/1 -> Product/2
  Actuator_State/1 -> Relational Operator/1
  Relational Operator/1 -> Switch/2

== system Twotanks_m71/Model/Environment/Sensor_HI_Tank2 ==
  current_height : Inport
  sensor_height : Inport  Port=2
  Constant : Constant  Value=0.0
  Constant1 : Constant  Value=1.0
  Relational Operator : RelationalOperator  Operator=>  OutDataTypeStr=boolean  RndMeth=Nearest
  Switch : Switch  Criteria=u2 ~= 0
  Sensor Value : Outport  VectorParamsAs1DForOutWhenUnconnected=off
  wires:
  Constant/1 -> Switch/1
  sensor_height/1 -> Relational Operator/1
  Constant1/1 -> Switch/3
  Relational Operator/1 -> Switch/2
  current_height/1 -> Relational Operator/2
  Switch/1 -> Sensor Value/1

== system Twotanks_m71/Model/Environment/Sensor_High_Tank1 ==
  current_height : Inport
  sensor_height : Inport  Port=2
  Constant : Constant  Value=0.0
  Constant1 : Constant  Value=1.0
  Relational Operator : RelationalOperator  Operator=>  OutDataTypeStr=boolean  RndMeth=Nearest
  Switch : Switch  Criteria=u2 ~= 0
  Sensor Value : Outport  VectorParamsAs1DForOutWhenUnconnected=off
  wires:
  Constant/1 -> Switch/1
  sensor_height/1 -> Relational Operator/1
  Constant1/1 -> Switch/3
  Relational Operator/1 -> Switch/2
  current_height/1 -> Relational Operator/2
  Switch/1 -> Sensor Value/1

== system Twotanks_m71/Model/Environment/Sensor_LO_Tank2 ==
  current_height : Inport
  sensor_height : Inport  Port=2
  Constant : Constant  Value=0.0
  Constant1 : Constant  Value=1.0
  Relational Operator : RelationalOperator  Operator=>  OutDataTypeStr=boolean  RndMeth=Nearest
  Switch : Switch  Criteria=u2 ~= 0
  Sensor Value : Outport  VectorParamsAs1DForOutWhenUnconnected=off
  wires:
  Constant/1 -> Switch/1
  Constant1/1 -> Switch/3
  Relational Operator/1 -> Switch/2
  Switch/1 -> Sensor Value/1
  current_height/1 -> Relational Operator/2
  sensor_height/1 -> Relational Operator/1

== system Twotanks_m71/Model/Environment/Sensor_Low_Tank1 ==
  current_height : Inport
  sensor_height : Inport  Port=2
  Constant : Constant  Value=0.0
  Constant1 : Constant  Value=1.0
  Relational Operator : RelationalOperator  Operator=>  OutDataTypeStr=boolean  RndMeth=Nearest
  Switch : Switch  Criteria=u2 ~= 0
  Sensor Value : Outport  VectorParamsAs1DForOutWhenUnconnected=off
  wires:
  Switch/1 -> Sensor Value/1
  current_height/1 -> Relational Operator/2
  Relational Operator/1 -> Switch/2
  Constant1/1 -> Switch/3
  sensor_height/1 -> Relational Operator/1
  Constant/1 -> Switch/1

== system Twotanks_m71/Model/Environment/Sensor_MD_Tank2 ==
  current_height : Inport
  sensor_height : Inport  Port=2
  Constant : Constant  Value=0.0
  Constant1 : Constant  Value=1.0
  Relational Operator : RelationalOperator  Operator=>  OutDataTypeStr=boolean  RndMeth=Nearest
  Switch : Switch  Criteria=u2 ~= 0
  Sensor Value : Outport  VectorParamsAs1DForOutWhenUnconnected=off
  wires:
  Switch/1 -> Sensor Value/1
  Relational Operator/1 -> Switch/2
  Constant1/1 -> Switch/3
  Constant/1 -> Switch/1
  current_height/1 -> Relational Operator/2
  sensor_height/1 -> Relational Operator/1

== system Twotanks_m71/Model/Environment/Tank1 ==
  previous_height_m : Inport
  pump_flow_rate_m3dt : Inport  Port=2
  cross_section_area_m2 : Inport  Port=3
  valve_flow_rate_m3dt : Inport  Port=4
  Divide : Product  Inputs=*/
  Sum : Sum  Inputs=|++
  Sum1 : Sum  Inputs=|+-
  liquid_height_m : Outport  VectorParamsAs1DForOutWhenUnconnected=off
  wires:
  previous_height_m/1 -> Sum/1
  Divide/1 -> Sum/2
  cross_section_area_m2/1 -> Divide/2
  Sum1/1 -> Divide/1
  valve_flow_rate_m3dt/1 -> Sum1/2
  pump_flow_rate_m3dt/1 -> Sum1/1
  Sum/1 -> liquid_height_m/1

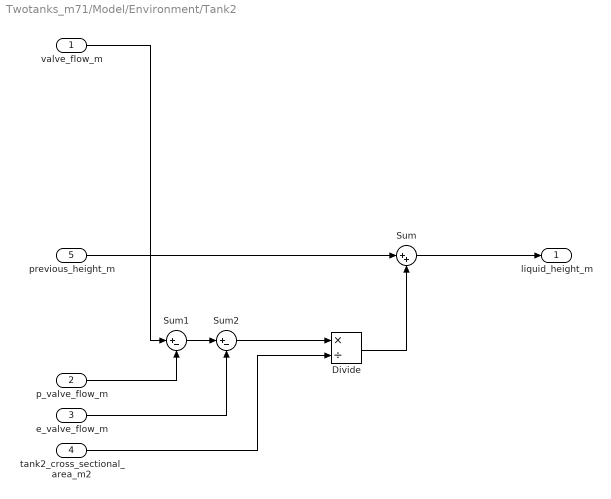
== system Twotanks_m71/Model/Environment/Tank2 ==
  valve_flow_m : Inport
  p_valve_flow_m : Inport  Port=2
  e_valve_flow_m : Inport  Port=3
  tank2_cross_sectional_area_m2 : Inport  Port=4
  previous_height_m : Inport  Port=5
  Divide : Product  Inputs=*/
  Sum : Sum  Inputs=|++
  Sum1 : Sum  Inputs=|+-
  Sum2 : Sum  Inputs=|+-
  liquid_height_m : Outport  VectorParamsAs1DForOutWhenUnconnected=off
  wires:
  e_valve_flow_m/1 -> Sum2/2
  Sum/1 -> liquid_height_m/1
  Divide/1 -> Sum/2
  tank2_cross_sectional_area_m2/1 -> Divide/2
  previous_height_m/1 -> Sum/1
  valve_flow_m/1 -> Sum1/1
  Sum2/1 -> Divide/1
  p_valve_flow_m/1 -> Sum1/2
  Sum1/1 -> Sum2/1

== system Twotanks_m71/Model/Environment/Valve ==
  Actuator_State : Inport
  actuator_flow_rate_m3s : Inport  Port=2
  time_increment1 : Inport  Port=3
  Constant1 : Constant  Value=0.0
  Constant2 : Constant  Value=0.5
  Product : Product
  Relational Operator : RelationalOperator  Operator=>  OutDataTypeStr=boolean  RndMeth=Nearest
  Switch : Switch  Criteria=u2 ~= 0
  flow_rate_m3dt : Outport  VectorParamsAs1DForOutWhenUnconnected=off
  wires:
  Relational Operator/1 -> Switch/2
  Actuator_State/1 -> Relational Operator/1
  time_increment1/1 -> Product/2
  Constant1/1 -> Switch/3
  Constant2/1 -> Relational Operator/2
  Switch/1 -> flow_rate_m3dt/1
  Product/1 -> Switch/1
  actuator_flow_rate_m3s/1 -> Product/1

== system Twotanks_m71/Model/Initializer_and_Updater/E_Valve_Initial_State ==
  initial_value : Inport
  Constant : Constant  Value=0.0
  Switch : Switch  Criteria=u2 > Threshold
  Unit Delay : UnitDelay  InitialCondition=1  SampleTime=-1  HasFrameUpgradeWarning=on
  Initial Value : Outport  VectorParamsAs1DForOutWhenUnconnected=off
  wires:
  Switch/1 -> Initial Value/1
  Constant/1 -> Switch/3, Unit Delay/1
  Unit Delay/1 -> Switch/2
  initial_value/1 -> Switch/1

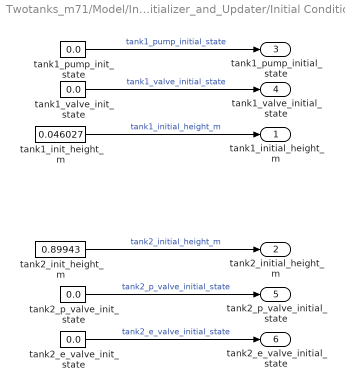
== system Twotanks_m71/Model/Initializer_and_Updater/Initial Conditions ==
  tank1_init_height_m : Constant  Value=0.046027
  tank1_pump_init_state : Constant  Value=0.0
  tank1_valve_init_state : Constant  Value=0.0
  tank2_e_valve_init_state : Constant  Value=0.0
  tank2_init_height_m : Constant  Value=0.89943
  tank2_p_valve_init_state : Constant  Value=0.0
  tank1_initial_height_m : Outport  VectorParamsAs1DForOutWhenUnconnected=off
  tank2_initial_height_m : Outport  Port=2  VectorParamsAs1DForOutWhenUnconnected=off
  tank1_pump_initial_state : Outport  Port=3  VectorParamsAs1DForOutWhenUnconnected=off
  tank1_valve_initial_state : Outport  Port=4  VectorParamsAs1DForOutWhenUnconnected=off
  tank2_p_valve_initial_state : Outport  Port=5  VectorParamsAs1DForOutWhenUnconnected=off
  tank2_e_valve_initial_state : Outport  Port=6  VectorParamsAs1DForOutWhenUnconnected=off
  wires:
  tank1_pump_init_state/1 -> tank1_pump_initial_state/1  "tank1_pump_initial_state"
  tank2_e_valve_init_state/1 -> tank2_e_valve_initial_state/1  "tank2_e_valve_initial_state"
  tank2_p_valve_init_state/1 -> tank2_p_valve_initial_state/1  "tank2_p_valve_initial_state"
  tank1_init_height_m/1 -> tank1_initial_height_m/1  "tank1_initial_height_m"
  tank2_init_height_m/1 -> tank2_initial_height_m/1  "tank2_initial_height_m"
  tank1_valve_init_state/1 -> tank1_valve_initial_state/1  "tank1_valve_initial_state"

== system Twotanks_m71/Model/Initializer_and_Updater/Initial_Height_Tank _2 ==
  initial_value : Inport
  Constant : Constant  Value=0.0
  Switch : Switch  Criteria=u2 > Threshold
  Unit Delay : UnitDelay  InitialCondition=1  SampleTime=-1  HasFrameUpgradeWarning=on
  Initial Value : Outport  VectorParamsAs1DForOutWhenUnconnected=off
  wires:
  Switch/1 -> Initial Value/1
  Constant/1 -> Switch/3, Unit Delay/1
  Unit Delay/1 -> Switch/2
  initial_value/1 -> Switch/1

== system Twotanks_m71/Model/Initializer_and_Updater/Initial_Height_Tank_1 ==
  initial_value : Inport
  Constant : Constant  Value=0.0
  Switch : Switch  Criteria=u2 > Threshold
  Unit Delay : UnitDelay  InitialCondition=1  SampleTime=-1  HasFrameUpgradeWarning=on
  Initial Value : Outport  VectorParamsAs1DForOutWhenUnconnected=off
  wires:
  Constant/1 -> Switch/3, Unit Delay/1
  Unit Delay/1 -> Switch/2
  initial_value/1 -> Switch/1
  Switch/1 -> Initial Value/1

== system Twotanks_m71/Model/Initializer_and_Updater/P_Valve_Initial_State ==
  initial_value : Inport
  Constant : Constant  Value=0.0
  Switch : Switch  Criteria=u2 > Threshold
  Unit Delay : UnitDelay  InitialCondition=1  SampleTime=-1  HasFrameUpgradeWarning=on
  Initial Value : Outport  VectorParamsAs1DForOutWhenUnconnected=off
  wires:
  Switch/1 -> Initial Value/1
  Constant/1 -> Switch/3, Unit Delay/1
  Unit Delay/1 -> Switch/2
  initial_value/1 -> Switch/1

== system Twotanks_m71/Model/Initializer_and_Updater/Pump_Initial_State ==
  initial_value : Inport
  Constant : Constant  Value=0.0
  Switch : Switch  Criteria=u2 > Threshold
  Unit Delay : UnitDelay  InitialCondition=1  SampleTime=-1  HasFrameUpgradeWarning=on
  Initial Value : Outport  VectorParamsAs1DForOutWhenUnconnected=off
  wires:
  Switch/1 -> Initial Value/1
  Constant/1 -> Switch/3, Unit Delay/1
  Unit Delay/1 -> Switch/2
  initial_value/1 -> Switch/1

== system Twotanks_m71/Model/Initializer_and_Updater/Valve_Initial_State ==
  initial_value : Inport
  Constant : Constant  Value=0.0
  Switch : Switch  Criteria=u2 > Threshold
  Unit Delay : UnitDelay  InitialCondition=1  SampleTime=-1  HasFrameUpgradeWarning=on
  Initial Value : Outport  VectorParamsAs1DForOutWhenUnconnected=off
  wires:
  Switch/1 -> Initial Value/1
  Constant/1 -> Switch/3, Unit Delay/1
  Unit Delay/1 -> Switch/2
  initial_value/1 -> Switch/1
